simulink model "fieldTest"  (R2023b)
settings: Solver=VariableStepAuto  StartTime=0.0  StopTime=40  RelTol=1e-3
values from neighbouring files (symbols this model uses):
  A = [-2.1979433138  -1.57242643331; 1  0]    [SinusDie1.mat]    (also in Test4.mat; Test5.mat)
  B = [1 0]    [SinusDie1.mat]    (also in Test4.mat; Test5.mat)
  C = [0 1.57242643331]    [SinusDie1.mat]    (also in Test4.mat; Test5.mat)
  data =     [SinusDie1.mat]    (also in Test4.mat; Test5.mat)
undefined symbols (not defined in the file or in its folder): National_Instruments, PCIe
libraries: sldrtlib x2, SignalEditorBlockLib x1
settings Model: Creator=ematric  LastModifiedBy=fluky
settings SolverCC: AlgebraicLoopSolver=TrustRegion
settings RTWCC: DLArmComputeVersion=19.05

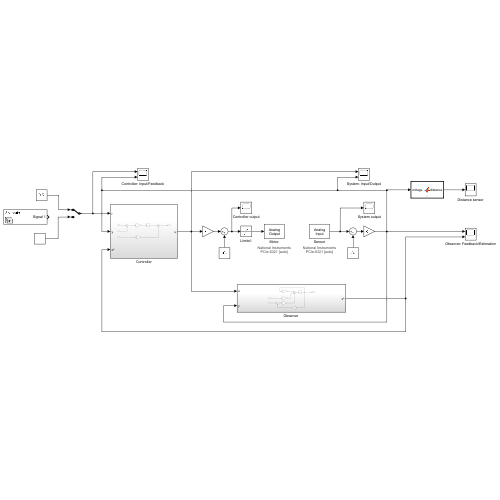
[thumbnail: Simulink's stored preview of the top-level diagram]
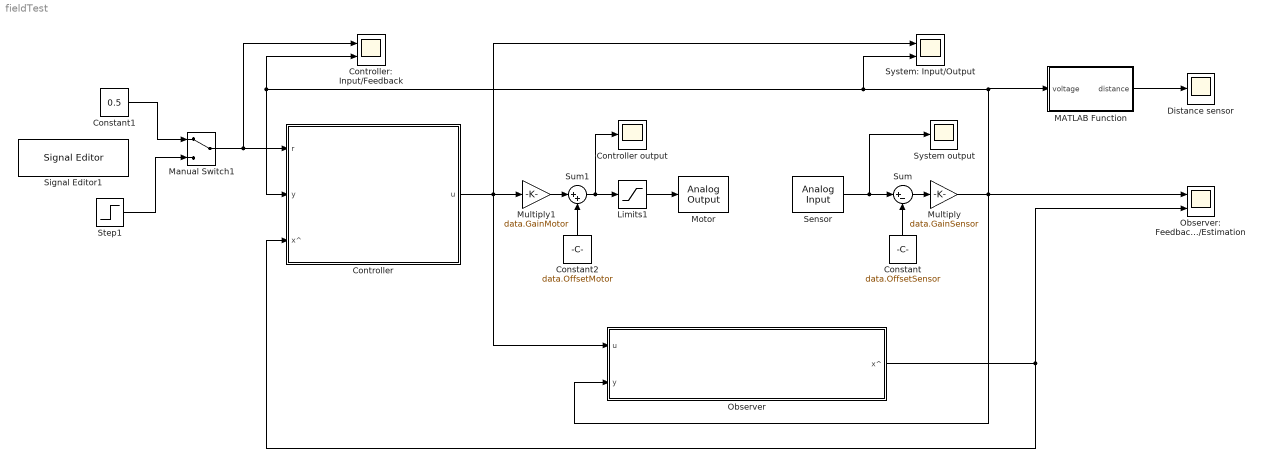
== system fieldTest ==
  Constant : Constant  Value=data.OffsetSensor
  Constant1 : Constant  Value=0.5
  Constant2 : Constant  Value=data.OffsetMotor
  Controller : Subsystem
  Controller output : Scope
  Controller: Input/Feedback : Scope  NumInputPorts=2
  Distance sensor : Scope
  Limits1 : Saturate  UpperLimit=5  LowerLimit=-5
  MATLAB Function : MATLAB Function  TreatAsAtomicUnit=on
  Manual Switch1 : ManualSwitch
  Motor : sldrtlib/Analog Output  SampleTime=0.1  MaxMissedTicks=10  ShowMissedTicks=off  YieldWhenWaiting=off  DrvName=National_Instruments/PCIe-6321  DrvAddress=4294967295  DrvOptions=[0 0 0 0 0 0 0]  Channels=1  RangeMode=1  VoltRange=1  InitialValue=0  FinalValue=0
      settings: AttributesFormatString=National Instruments\nPCIe-6321 [auto]
  Multiply : Gain  Gain=data.GainSensor
  Multiply1 : Gain  Gain=data.GainMotor
  "Observer " : Subsystem
  Observer: Feedback/Estimation : Scope  NumInputPorts=2
  Sensor : sldrtlib/Analog Input  SampleTime=0.1  MaxMissedTicks=10  ShowMissedTicks=off  YieldWhenWaiting=off  DrvName=National_Instruments/PCIe-6321  DrvAddress=4294967295  DrvOptions=[0 0 0 0 0 0 0]  Channels=1  RangeMode=1  VoltRange=1  DataType=1
      settings: AttributesFormatString=National Instruments\nPCIe-6321 [auto]
  Signal Editor1 : SignalEditorBlockLib/Signal Editor  FileName=trajectories.mat  ActiveScenario=Scenario  ActiveSignal=TestSignal  IsBus=off  OutputBusObjectStr=Bus: BusObject  SampleTime=0  Interpolate=off  ZeroCross=off  OutputAfterFinalValue=Setting to zero  Unit=inherit  PreserveSignalName=on  ApplySigPropsToAllScenarios=on  ApplySigPropsToAllSignals=off
  Step1 : Step  Time=0  SampleTime=0
  Sum : Sum  Inputs=|+-
  Sum1 : Sum  Inputs=|++
  System output : Scope
  System: Input/Output : Scope  NumInputPorts=2
  wires:
  "Observer "/1(x^) -> Controller/3(x^), Observer: Feedback/Estimation/2
  Step1/1 -> Manual Switch1/2
  Manual Switch1/1 -> Controller: Input/Feedback/1, Controller/1(r)
  Sum/1 -> Multiply/1
  MATLAB Function/1(distance) -> Distance sensor/1
  Sensor/1 -> System output/1, Sum/1
  Constant/1 -> Sum/2
  Multiply/1 -> Observer: Feedback/Estimation/1, System: Input/Output/2, Controller/2(y), Controller: Input/Feedback/2, MATLAB Function/1(voltage), "Observer "/2(y)
  Constant1/1 -> Manual Switch1/1
  Constant2/1 -> Sum1/2
  Controller/1(u) -> Multiply1/1, System: Input/Output/1, "Observer "/1(u)
  Multiply1/1 -> Sum1/1
  Sum1/1 -> Limits1/1, Controller output/1
  Limits1/1 -> Motor/1

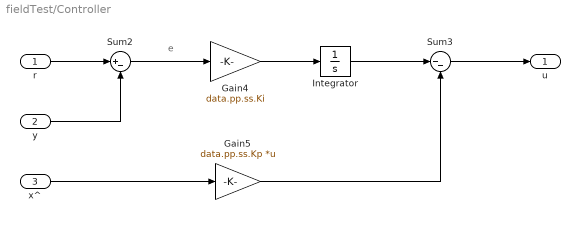
== system fieldTest/Controller ==
  note: e
  r : Inport
  y : Inport  Port=2
  x^ : Inport  Port=3
  Gain4 : Gain  Gain=data.pp.ss.Ki
  Gain5 : Gain  Gain=data.pp.ss.Kp  Multiplication=Matrix(K*u)
  Integrator : Integrator
  Sum2 : Sum  Inputs=|+-
  Sum3 : Sum  Inputs=|--
  u : Outport
  wires:
  Integrator/1 -> Sum3/1
  Gain4/1 -> Integrator/1
  Sum2/1 -> Gain4/1
  Gain5/1 -> Sum3/2
  r/1 -> Sum2/1
  y/1 -> Sum2/2
  Sum3/1 -> u/1
  x^/1 -> Gain5/1

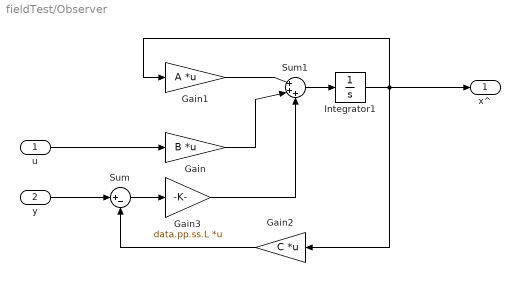
== system fieldTest/Observer  ==
  u : Inport
  y : Inport  Port=2
  Gain : Gain  Gain=B  Multiplication=Matrix(K*u)
  Gain1 : Gain  Gain=A  Multiplication=Matrix(K*u)
  Gain2 : Gain  Gain=C  Multiplication=Matrix(K*u)
  Gain3 : Gain  Gain=data.pp.ss.L  Multiplication=Matrix(K*u)
  Integrator1 : Integrator
  Sum : Sum  Inputs=|+-
  Sum1 : Sum  Inputs=|+++
  x^ : Outport
  wires:
  Gain1/1 -> Sum1/1
  Gain2/1 -> Sum/2
  Sum/1 -> Gain3/1
  Integrator1/1 -> x^/1, Gain2/1, Gain1/1
  Gain/1 -> Sum1/2
  Gain3/1 -> Sum1/3
  Sum1/1 -> Integrator1/1
  u/1 -> Gain/1
  y/1 -> Sum/1

== matlab function fieldTest/MATLAB Function ==
  data: voltage input; distance output
function distance = fcn(voltage)

distance=(73.3604*voltage.^3)+(-339.1311*voltage.^2)+(527.2338*voltage)+(-242.9424);
